simulink model "dummy"  (R2017b)
settings: Solver=VariableStepAuto  StartTime=0.0  StopTime=10.0  MaxStep=0.001  RelTol=1e-3
settings Model: Creator=user  LastModifiedBy=user

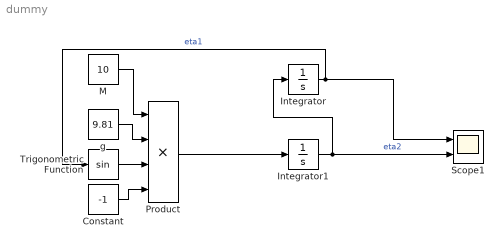
== system dummy ==
  Constant : Constant  Value=-1
  Integrator : Integrator  InitialCondition=1e-2
  Integrator1 : Integrator
  M : Constant  Value=10
  Product : Product  Inputs=4
  Scope1 : Scope  NumInputPorts=2
  Trigonometric Function : Trigonometry
  g : Constant  Value=9.81
  wires:
  Integrator1/1 -> Integrator/1, Scope1/2  "eta2"
  Integrator/1 -> Scope1/1, Trigonometric Function/1  "eta1"
  Trigonometric Function/1 -> Product/3
  Product/1 -> Integrator1/1
  Constant/1 -> Product/4
  g/1 -> Product/2
  M/1 -> Product/1
